simulink model "pendule_inv_echant_etu"  (R2019a)
settings: Solver=VariableStepAuto  StartTime=0.0  StopTime=tf  RelTol=1e-3
values from neighbouring files (symbols this model uses):
  delta_t = 0.1    [simu_pendule_inv_echant_etu.m]
  g = 9.81    [simu_pendule_inv_capteur_etu.m]    (also in simu_pendule_inv_echant_etu.m)
  K = [10 1]    [simu_pendule_inv_capteur_etu.m]    (also in simu_pendule_inv_echant_etu.m = [30 10])
  l = 10    [simu_pendule_inv_capteur_etu.m]    (also in simu_pendule_inv_echant_etu.m)
  ue = 0    [simu_pendule_inv_capteur_etu.m]    (also in simu_pendule_inv_echant_etu.m)
  x0 = [pi/20 0]'    [simu_pendule_inv_capteur_etu.m]    (also in simu_pendule_inv_echant_etu.m)
  xe = [0 0]'    [simu_pendule_inv_capteur_etu.m]    (also in simu_pendule_inv_echant_etu.m)
undefined symbols (not defined in the file or in its folder): DiscIntNeverNeededParam
settings Model: Creator=nravalos  LastModifiedBy=nravalos

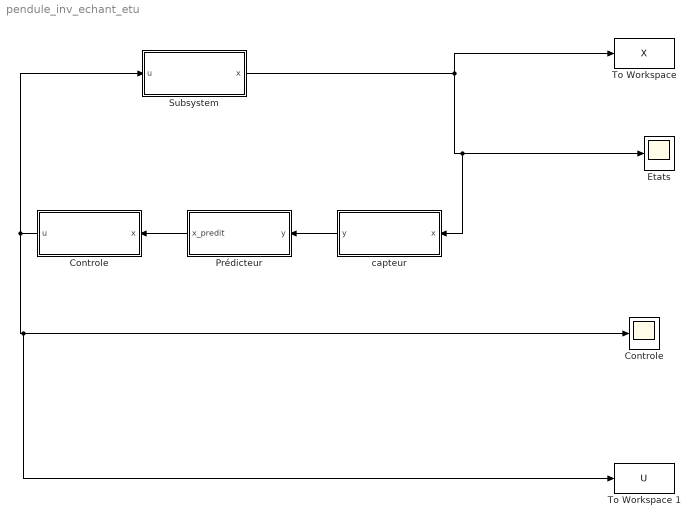
== system pendule_inv_echant_etu ==
  Controle : Subsystem
  "Controle " : Scope
  Etats : Scope
  "Prédicteur " : Subsystem
  Subsystem : Subsystem
  "To Workspace " : ToWorkspace  VariableName=X  SaveFormat=Timeseries  SampleTime=-1
  "To Workspace 1 " : ToWorkspace  VariableName=U  SaveFormat=Timeseries  SampleTime=-1
  capteur : Subsystem
  wires:
  Controle/1(u) -> Subsystem/1("u "), "To Workspace 1 "/1, "Controle "/1
  capteur/1("y ") -> "Prédicteur "/1("y ")
  "Prédicteur "/1("x_predit ") -> Controle/1(x)
  Subsystem/1(x) -> capteur/1("x "), Etats/1, "To Workspace "/1

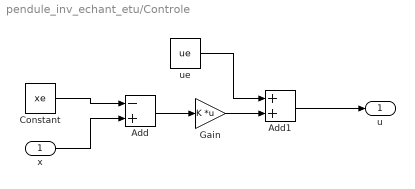
== system pendule_inv_echant_etu/Controle ==
  x : Inport
  Add : Sum  Inputs=-+
  Add1 : Sum
  Constant : Constant  Value=xe
  Gain : Gain  Gain=K  Multiplication=Matrix(K*u)
  ue : Constant  Value=ue
  u : Outport
  wires:
  x/1 -> Add/2
  Add1/1 -> u/1
  ue/1 -> Add1/1
  Gain/1 -> Add1/2
  Constant/1 -> Add/1
  Add/1 -> Gain/1

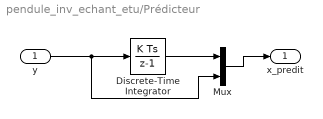
== system pendule_inv_echant_etu/Prédicteur  ==
  "y " : Inport
  Discrete-Time Integrator : DiscreteIntegrator  InitialCondition=x0(1)  SampleTime=-1  ICPrevOutput=DiscIntNeverNeededParam  ICPrevScaledInput=DiscIntNeverNeededParam
  Mux : Mux  Inputs=2
  "x_predit " : Outport
  wires:
  "y "/1 -> Discrete-Time Integrator/1, Mux/2
  Discrete-Time Integrator/1 -> Mux/1
  Mux/1 -> "x_predit "/1

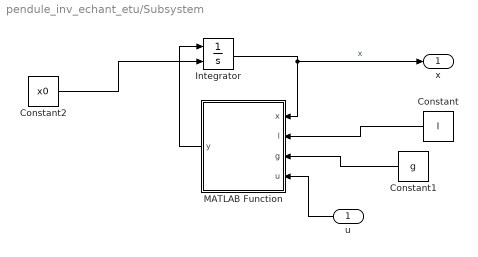
== system pendule_inv_echant_etu/Subsystem ==
  "u " : Inport
  Constant : Constant  Value=l
  Constant1 : Constant  Value=g
  Constant2 : Constant  Value=x0
  Integrator : Integrator  InitialConditionSource=external
  MATLAB Function : MATLAB Function  TreatAsAtomicUnit=on
  x : Outport
  wires:
  "u "/1 -> MATLAB Function/4(u)
  Integrator/1 -> MATLAB Function/1(x), x/1  "x"
  MATLAB Function/1(y) -> Integrator/1
  Constant/1 -> MATLAB Function/2(l)
  Constant1/1 -> MATLAB Function/3(g)
  Constant2/1 -> Integrator/2

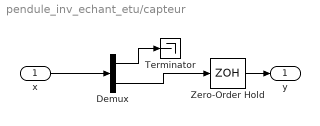
== system pendule_inv_echant_etu/capteur ==
  "x " : Inport
  Demux : Demux  Outputs=2
  Terminator : Terminator
  Zero-Order Hold : ZeroOrderHold  SampleTime=delta_t
  "y " : Outport
  wires:
  "x "/1 -> Demux/1
  Demux/2 -> Zero-Order Hold/1
  Demux/1 -> Terminator/1
  Zero-Order Hold/1 -> "y "/1

== matlab function pendule_inv_echant_etu/Subsystem/MATLAB Function ==
  data: x input; l input; g input; u input; y output
function y = fcn(x, l, g, u)

y=[x(2),(g/l)*sin(x(1))-cos(x(1))*u/l];
